simulink model "System"  (R2021b)
settings: Solver=VariableStepAuto  StartTime=0.0  StopTime=10.0  RelTol=1e-3
model workspace (MAT data in the model file):
  A = 1
  B = 1
  C = 1
  Q1 = 0.02
  Q2 = 0.05
  R = 0.05
  alp = 0.001
  bet = 2
  ki = 0
libraries: matrix_library x2, dspmtrx3 x1
settings Model: Creator=aakas  LastModifiedBy=aakas

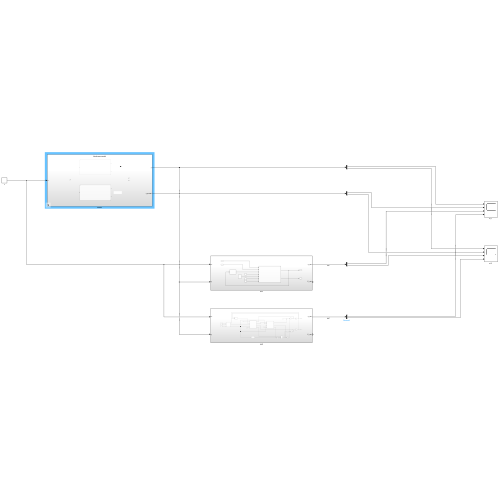
[thumbnail: Simulink's stored preview of the top-level diagram]
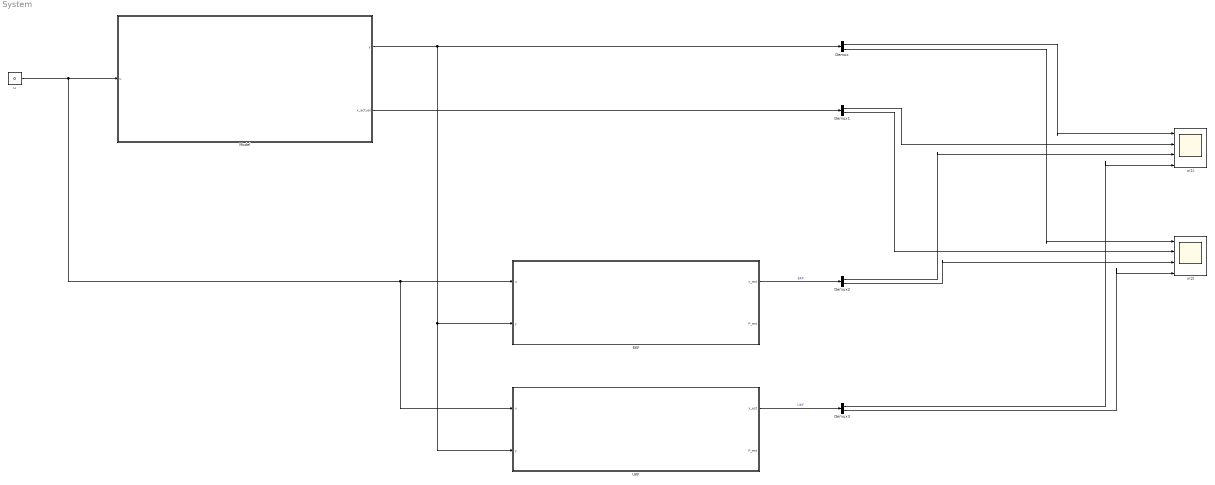
== system System ==
  Demux{,1..3} (4 alike) : Demux  Outputs=2
  EKF : Subsystem
  Model : Subsystem  Variant=on  VariantControlMode=label  VariantControl=Choice  LabelModeActiveChoice=Choice
  UKF : Subsystem
  u : Constant  Value=0
  x(1) : Scope  NumInputPorts=4
  x(2) : Scope  NumInputPorts=4
  wires:
  u/1 -> EKF/1(u), UKF/1(u), Model/1(u)
  Model/1(y) -> UKF/2(y), EKF/2(y), Demux/1
  Model/2(x_actual) -> Demux1/1
  Demux/2 -> x(2)/1
  Demux/1 -> x(1)/1
  Demux1/1 -> x(1)/2
  Demux1/2 -> x(2)/2
  EKF/1(x_est) -> Demux2/1  "EKF"
  Demux2/1 -> x(1)/3
  Demux2/2 -> x(2)/3
  UKF/1(x_est) -> Demux3/1  "UKF"
  Demux3/1 -> x(1)/4
  Demux3/2 -> x(2)/4

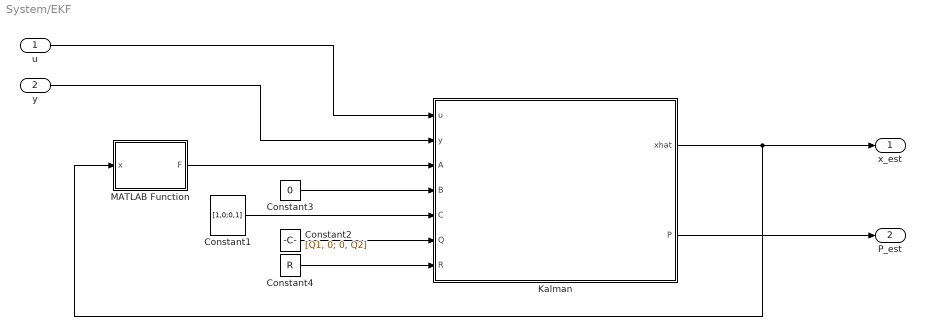
== system System/EKF ==
  u : Inport
  y : Inport  Port=2
  Constant1 : Constant  Value=[1,0;0,1]  VectorParams1D=off
  Constant2 : Constant  Value=[Q1, 0; 0, Q2]
  Constant3 : Constant  Value=0
  Constant4 : Constant  Value=R
  Kalman : Subsystem
  MATLAB Function : MATLAB Function  TreatAsAtomicUnit=on
  x_est : Outport
  P_est : Outport  Port=2
  wires:
  u/1 -> Kalman/1(u)
  y/1 -> Kalman/2(y)
  Constant3/1 -> Kalman/4(B)
  Constant1/1 -> Kalman/5(C)
  Kalman/1(xhat) -> x_est/1, MATLAB Function/1(x)
  Constant2/1 -> Kalman/6(Q)
  Constant4/1 -> Kalman/7(R)
  MATLAB Function/1(F) -> Kalman/3(A)
  Kalman/2(P) -> P_est/1

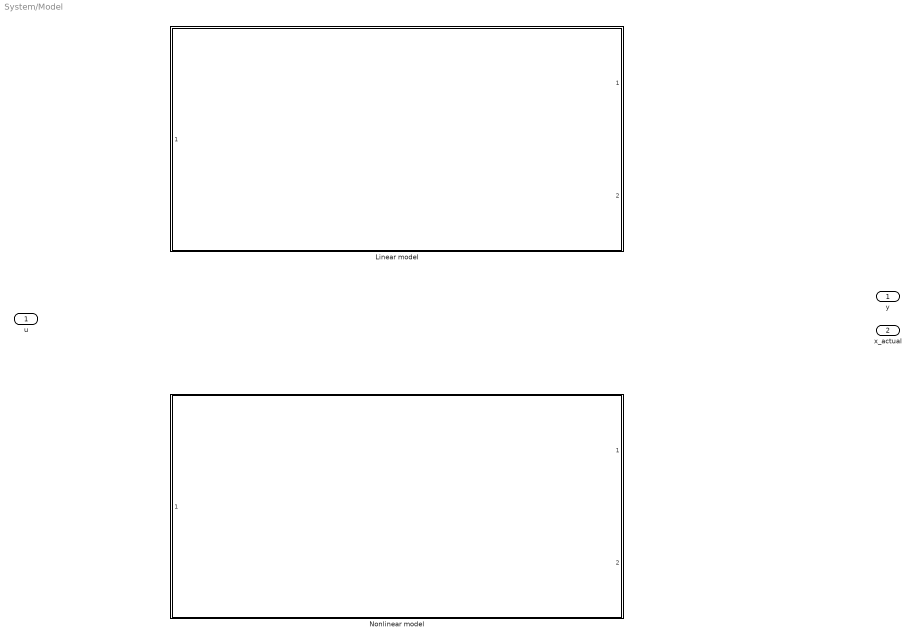
== system System/Model ==
  u : Inport
  Linear model : Subsystem  VariantControl=Choice_1  ReferencedSubsystem=Linear_model
  Nonlinear model : Subsystem  VariantControl=Choice  ReferencedSubsystem=Nonlinear_model
  y : Outport
  x_actual : Outport  Port=2

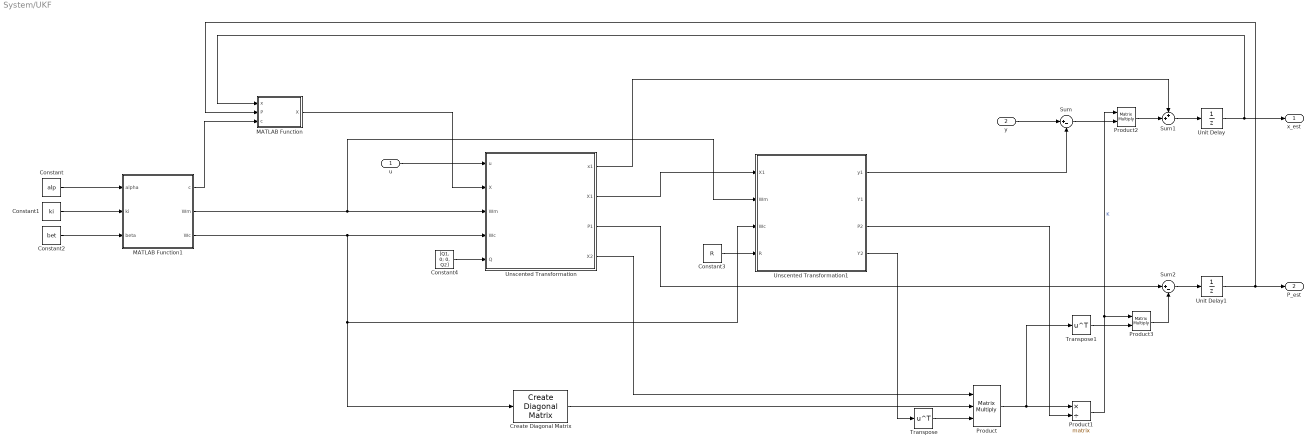
== system System/UKF ==
  u : Inport
  y : Inport  Port=2
  Constant : Constant  Value=alp
  Constant1 : Constant  Value=ki
  Constant2 : Constant  Value=bet
  Constant3 : Constant  Value=R
  Constant4 : Constant  Value=[Q1, 0; 0, Q2]
  Create Diagonal Matrix : dspmtrx3/Create Diagonal Matrix
      settings: SourceProductBaseCode=DS
  MATLAB Function : MATLAB Function  TreatAsAtomicUnit=on
  MATLAB Function1 : MATLAB Function  TreatAsAtomicUnit=on
  Product : Product  Inputs=3  Multiplication=Matrix(*)
  Product1 : Product  Inputs=*/  Multiplication=Matrix(*)
  Product2 : Product  Multiplication=Matrix(*)
  Product3 : Product  Multiplication=Matrix(*)
  Sum : Sum  Inputs=|+-
  Sum1 : Sum  Inputs=++|
  Sum2 : Sum  Inputs=|+-
  Transpose : Math  Operator=transpose  SaturateOnIntegerOverflow=on
  Transpose1 : Math  Operator=transpose  SaturateOnIntegerOverflow=on
  Unit Delay : UnitDelay  InitialCondition=[1; 0]  SampleTime=-1  HasFrameUpgradeWarning=on
  Unit Delay1 : UnitDelay  InitialCondition=[1, 0; 0, 0.1]  SampleTime=-1  HasFrameUpgradeWarning=on
  Unscented Transformation : MATLAB Function  TreatAsAtomicUnit=on
  Unscented Transformation1 : MATLAB Function  TreatAsAtomicUnit=on
  x_est : Outport
  P_est : Outport  Port=2
  wires:
  Constant/1 -> MATLAB Function1/1(alpha)
  Constant1/1 -> MATLAB Function1/2(ki)
  MATLAB Function1/1(c) -> MATLAB Function/3(c)
  Constant4/1 -> Unscented Transformation/5(Q)
  MATLAB Function/1(X) -> Unscented Transformation/2(X)
  Constant2/1 -> MATLAB Function1/3(beta)
  MATLAB Function1/2(Wm) -> Unscented Transformation1/2(Wm), Unscented Transformation/3(Wm)
  MATLAB Function1/3(Wc) -> Create Diagonal Matrix/1, Unscented Transformation1/3(Wc), Unscented Transformation/4(Wc)
  Unscented Transformation/2(X1) -> Unscented Transformation1/1(X1)
  Constant3/1 -> Unscented Transformation1/4(R)
  Unscented Transformation/4(X2) -> Product/1
  Create Diagonal Matrix/1 -> Product/2
  Transpose/1 -> Product/3
  y/1 -> Sum/1
  Unscented Transformation1/1(y1) -> Sum/2
  Sum/1 -> Product2/2
  Product/1 -> Product1/1, Transpose1/1
  Product1/1 -> Product3/1, Product2/1  "K"
  Product2/1 -> Sum1/2
  Unscented Transformation/1(x1) -> Sum1/1
  Sum1/1 -> Unit Delay/1
  Unit Delay/1 -> x_est/1, MATLAB Function/1(x)
  Transpose1/1 -> Product3/2
  Unscented Transformation/3(P1) -> Sum2/1
  Product3/1 -> Sum2/2
  Sum2/1 -> Unit Delay1/1
  Unit Delay1/1 -> P_est/1, MATLAB Function/2(P)
  u/1 -> Unscented Transformation/1(u)
  Unscented Transformation1/3(P2) -> Product1/2
  Unscented Transformation1/4(Y2) -> Transpose/1

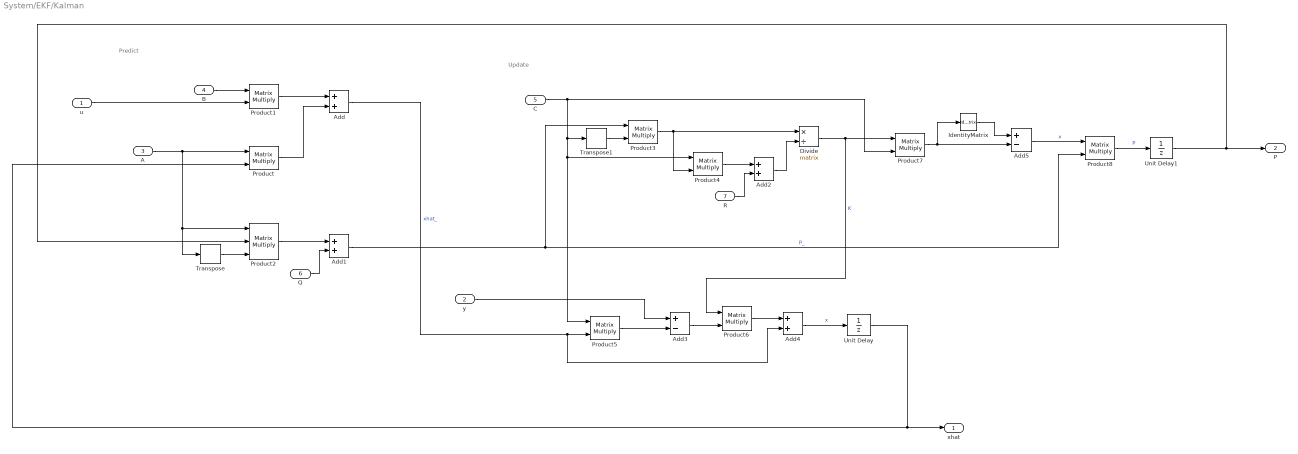
== system System/EKF/Kalman ==
  note: Predict
  note: Update
  u : Inport
  y : Inport  Port=2
  A : Inport  Port=3
  B : Inport  Port=4
  C : Inport  Port=5
  Q : Inport  Port=6
  R : Inport  Port=7
  Add{,1..2,4} (4 alike) : Sum
  Add3 : Sum  Inputs=+-
  Add5 : Sum  Inputs=+-
  Divide : Product  Inputs=*/  Multiplication=Matrix(*)
  IdentityMatrix : IdentityMatrix  InheritOutputPortAttributes=on
  Product{,1,3..8} (8 alike) : Product  Inputs=**  Multiplication=Matrix(*)
  Product2 : Product  Inputs=***  Multiplication=Matrix(*)
  Transpose : matrix_library/Transpose
      settings: SourceProductBaseCode=SL
  Transpose1 : matrix_library/Transpose
      settings: SourceProductBaseCode=SL
  Unit Delay : UnitDelay  InitialCondition=[1; 0]  SampleTime=-1  HasFrameUpgradeWarning=on
  Unit Delay1 : UnitDelay  InitialCondition=[1, 0; 0, 0.1]  SampleTime=-1  HasFrameUpgradeWarning=on
  xhat : Outport
  P : Outport  Port=2
  wires:
  Product8/1 -> Unit Delay1/1  "P"
  y/1 -> Add3/1
  Add1/1 -> Product3/1, Product8/2  "P_"
  Divide/1 -> Product7/1, Product6/1  "K"
  Add/1 -> Add4/2, Product5/2  "xhat_"
  C/1 -> Product5/1, Product4/1, Transpose1/1, Product7/2
  Product3/1 -> Divide/1, Product4/2
  Add2/1 -> Divide/2
  IdentityMatrix/1 -> Add5/1
  Add3/1 -> Product6/2
  Product7/1 -> Add5/2, IdentityMatrix/1
  Transpose1/1 -> Product3/2
  Product4/1 -> Add2/1
  Product1/1 -> Add/1
  Product6/1 -> Add4/1
  Add4/1 -> Unit Delay/1  "x"
  A/1 -> Product/1, Product2/1, Transpose/1
  Product/1 -> Add/2
  Transpose/1 -> Product2/3
  B/1 -> Product1/1
  Product2/1 -> Add1/1
  R/1 -> Add2/2
  u/1 -> Product1/2
  Q/1 -> Add1/2
  Product5/1 -> Add3/2
  Add5/1 -> Product8/1  "x"
  Unit Delay/1 -> xhat/1, Product/2
  Unit Delay1/1 -> P/1, Product2/2

== matlab function System/EKF/MATLAB Function ==
  data: x input; F output
function F = dfdx(x)

F = [0, 1; -2*x(1)*x(2) - 1, 1-x(1)^2];

== matlab function System/UKF/MATLAB Function ==
  data: x input; X output; P input; c input
function X = sigmas(x,P,c)

A = c*chol(P)';
Y = x(:,ones(1,numel(x)));
X = [x Y+A Y-A];

== matlab function System/UKF/Unscented Transformation ==
  data: u input; X input; Wm input; Wc input; Q input; x1 output; X1 output; P1 output; X2 output
function [x1,X1,P1,X2] = ut1(u,X,Wm,Wc,Q)

n=2;
f = @(x,u) [x(2); (1-x(1)^2)*x(2)-x(1)];
L=size(X,2);
x1=zeros(n,1);
X1=zeros(n,L);
for k=1:L                   
    X1(:,k)=f(X(:,k),u);       
    x1=x1+Wm(k)*X1(:,k);       
end
X2=X1-x1(:,ones(1,L));
P1=X2*diag(Wc)*X2'+Q;

== matlab function System/UKF/MATLAB Function1 ==
  data: alpha input; ki input; beta input; c output; Wm output; Wc output
function [c,Wm,Wc] = weights(alpha, ki, beta)

L=2;
lambda=alpha^2*(L+ki)-L;
c=L+lambda;
Wm=[lambda/c 0.5/c+zeros(1,2*L)];
Wc=Wm;
Wc(1)=Wc(1)+(1-alpha^2+beta);
c=sqrt(c);

== matlab function System/UKF/Unscented Transformation1 ==
  data: X1 input; Wm input; Wc input; y1 output; Y1 output; R input; P2 output; Y2 output
function [y1,Y1,P2,Y2] = ut(X1,Wm,Wc,R)

n=2;
g = @(x) x;
L=size(X1,2);
y1=zeros(n,1);
Y1=zeros(n,L);
for k=1:L                   
    Y1(:,k)=g(X1(:,k));       
    y1=y1+Wm(k)*Y1(:,k);       
end
Y2=Y1-y1(:,ones(1,L));
P2=Y2*diag(Wc)*Y2'+R;
